simulink model "FCS"  (R2021a)
settings: Solver=VariableStepAuto  StartTime=0.0  StopTime=10.0  RelTol=1e-3
settings Model: Creator=mario  LastModifiedBy=mario
settings SolverCC: AlgebraicLoopSolver=TrustRegion
settings DataIOCC: ReturnWorkspaceOutputs=off
settings DebuggingCC: SFMachineParentedDataDiag=warning  ArithmeticOperatorsInVariantConditions=warning
settings SFSimCC: CustomCodeUndefinedFunction=UseInterfaceOnly

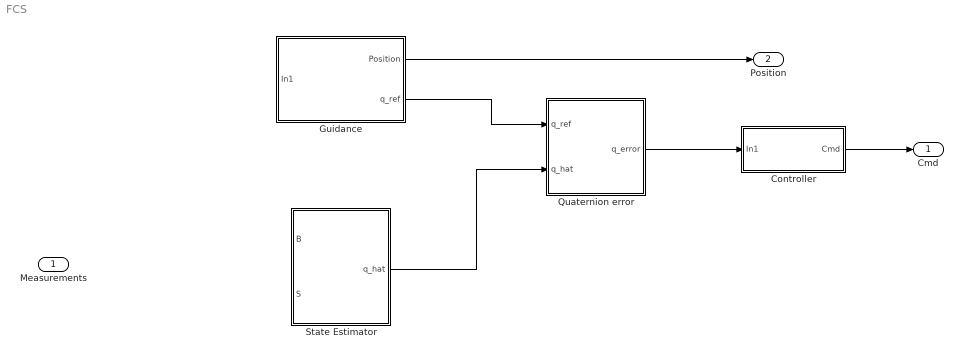
== system FCS ==
  Measurements : Inport
  Controller : Subsystem
  Guidance : Subsystem
  Quaternion error : Subsystem
  State Estimator : Subsystem
  Cmd : Outport  VectorParamsAs1DForOutWhenUnconnected=off
  Position : Outport  Port=2  VectorParamsAs1DForOutWhenUnconnected=off
  wires:
  Quaternion error/1(q_error) -> Controller/1(In1)
  Controller/1(Cmd) -> Cmd/1
  Guidance/1(Position) -> Position/1
  State Estimator/1(q_hat) -> Quaternion error/2(q_hat)
  Guidance/2(q_ref) -> Quaternion error/1(q_ref)

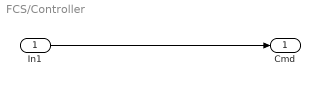
== system FCS/Controller ==
  In1 : Inport
  Cmd : Outport  VectorParamsAs1DForOutWhenUnconnected=off
  wires:
  In1/1 -> Cmd/1

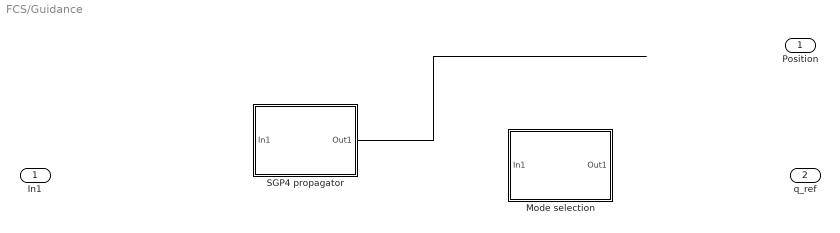
== system FCS/Guidance ==
  In1 : Inport
  Mode selection : Subsystem
  SGP4 propagator : Subsystem
  Position : Outport
  q_ref : Outport  Port=2
  wires:
  SGP4 propagator/1(Out1) -> ?

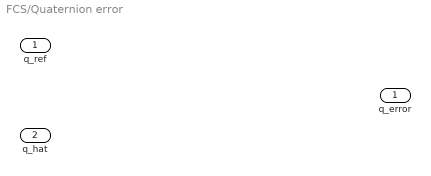
== system FCS/Quaternion error ==
  q_ref : Inport
  q_hat : Inport  Port=2
  q_error : Outport

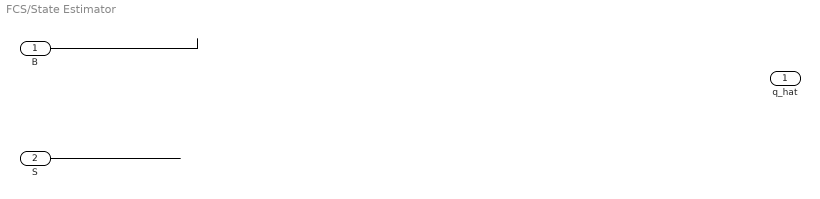
== system FCS/State Estimator ==
  B : Inport
  S : Inport  Port=2
  q_hat : Outport  VectorParamsAs1DForOutWhenUnconnected=off
  wires:
  B/1 -> ?
  S/1 -> ?

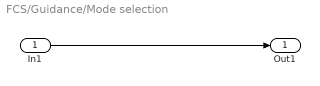
== system FCS/Guidance/Mode selection ==
  In1 : Inport
  Out1 : Outport
  wires:
  In1/1 -> Out1/1

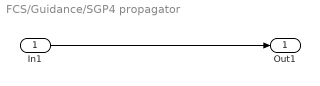
== system FCS/Guidance/SGP4 propagator ==
  In1 : Inport
  Out1 : Outport
  wires:
  In1/1 -> Out1/1
